simulink model "sedemo_preempt_policy"  (Simulink 7.5)
settings: Solver=VariableStepDiscrete  StartTime=0.0  StopTime=15  MaxStep=inf  RelTol=1e-3
libraries: simeventssink1 x10, simeventsgenerators1 x6, simeventsqueue1 x3, simeventsattributes2 x3, simeventsserver1 x3, simeventsprobes1 x2, simeventsrouting1 x2
settings Model: Creator=The MathWorks Inc.  ExtModeAutoUpdateStatusClock=off
settings DataIOCC: SaveOutput=off  SaveTime=off
settings OptimizationCC: InitFltsAndDblsToZero=on
settings DebuggingCC: AlgebraicLoopMsg=error  SaveWithParameterizedLinksMsg=none  SignalResolutionControl=TryResolveAllWithWarning  SolverPrmCheckMsg=none  MultiTaskDSMMsg=warning  MultiTaskCondExecSysMsg=none  StrictBusMsg=Warning
settings RTWCC: IncludeERTFirstTime=on
settings GRTTargetCC: TargetFcnLib=ansi_tfl_tmw.mat
settings SimEventsCC: propIdentEventSeed=12345678  propDiagAttribOutput=1  propDiagFcnCallOutput=1  propDiagStatOutput=0  propRNGIdenticalSeeds=0

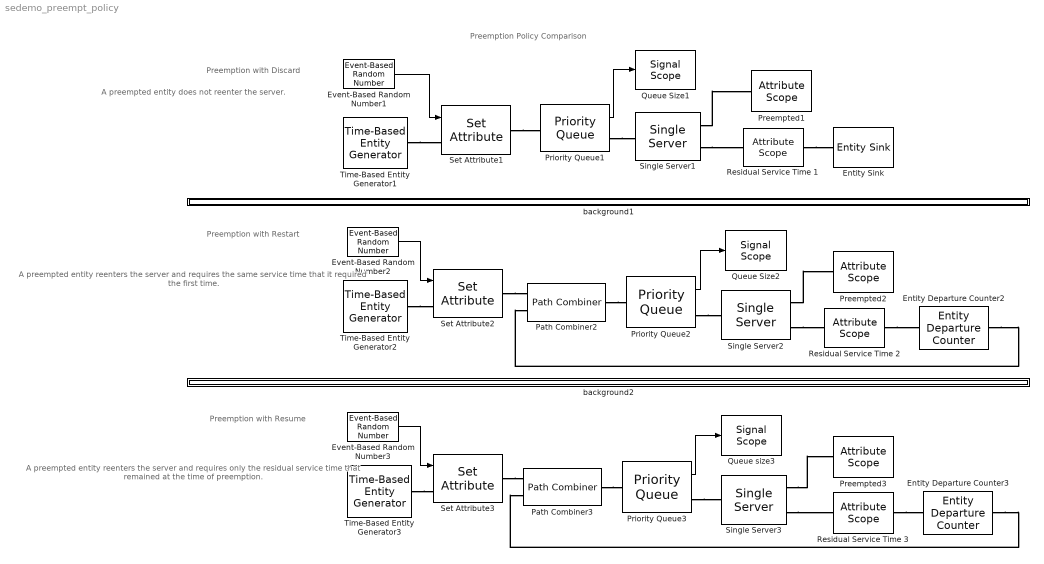
== system sedemo_preempt_policy ==
  note: Preemption with Restart
  note: Preemption with Resume
  note: A preempted entity does
      | not reenter the server.
  note: Preemption with Discard
  note: Preemption Policy Comparison
  note: A preempted entity reenters
      | the server and requires the
      | same service time that it
      | required the first time.
  note: A preempted entity reenters
      | the server and requires only
      | the residual service time
      | that remained at the time
      | of preemption.
  Entity Departure Counter2 : simeventsprobes1/Entity Departure Counter  Priority=1  SystemSampleTime=-1  NumberDepartedToSignal=Off  NumberDepartedToAttribute=On  NumberDepartedAttributeName=Preempted  CreateAttribute=on  CounterResetTypeOption=Off  CounterResetEdgeOption=Rising  SpecifyEventPriority=off  PriorityEntityCounterReset=1
  Entity Departure Counter3 : simeventsprobes1/Entity Departure Counter  Priority=1  SystemSampleTime=-1  NumberDepartedToSignal=Off  NumberDepartedToAttribute=On  NumberDepartedAttributeName=Preempted  CreateAttribute=on  CounterResetTypeOption=Off  CounterResetEdgeOption=Rising  SpecifyEventPriority=off  PriorityEntityCounterReset=1
  Entity Sink : simeventssink1/Entity Sink  Priority=1  SystemSampleTime=-1  AvailableForArrivals=on  StatNumberArrived=Off
  Event-Based Random Number1 : simeventsgenerators1/Signal Generators/Event-Based Random Number  SystemSampleTime=-1  distribution=Arbitrary discrete  meanExp=1  minUnif=0  maxUnif=1  pOneBern=0.25  pSuccessBino=0.5  numTrialBino=1  meanNorm=0  stdNorm=1  minTri=1  maxTri=3  modeTri=2  thresholdLogn=0  scaleLogn=1  shapeLogn=1  pSuccessGeo=0.5  meanPoiss=1  thresholdLogl=0  scaleLogl=1  thresholdGam=0  scaleGam=1  shapeGam=1  minBeta=0  maxBeta=1  shape1Beta=1  shape2Beta=1  minUnid=0  maxUnid=1  numValueUnid=2  thresholdWbl=0  scaleWbl=1  shapeWbl=1  valueVecCont=[0 1]  cdfVecCont=[0 1]  valueVecDisc=[1 2]  probVecDisc=[0.3 0.7]  seed=12345  IsProcessed=on  isConnected=1
  Event-Based Random Number2 : simeventsgenerators1/Signal Generators/Event-Based Random Number  SystemSampleTime=-1  distribution=Arbitrary discrete  meanExp=1  minUnif=0  maxUnif=1  pOneBern=0.25  pSuccessBino=0.5  numTrialBino=1  meanNorm=0  stdNorm=1  minTri=1  maxTri=3  modeTri=2  thresholdLogn=0  scaleLogn=1  shapeLogn=1  pSuccessGeo=0.5  meanPoiss=1  thresholdLogl=0  scaleLogl=1  thresholdGam=0  scaleGam=1  shapeGam=1  minBeta=0  maxBeta=1  shape1Beta=1  shape2Beta=1  minUnid=0  maxUnid=1  numValueUnid=2  thresholdWbl=0  scaleWbl=1  shapeWbl=1  valueVecCont=[0 1]  cdfVecCont=[0 1]  valueVecDisc=[1 2]  probVecDisc=[0.3 0.7]  seed=12345  IsProcessed=on  isConnected=1
  Event-Based Random Number3 : simeventsgenerators1/Signal Generators/Event-Based Random Number  SystemSampleTime=-1  distribution=Arbitrary discrete  meanExp=1  minUnif=0  maxUnif=1  pOneBern=0.25  pSuccessBino=0.5  numTrialBino=1  meanNorm=0  stdNorm=1  minTri=1  maxTri=3  modeTri=2  thresholdLogn=0  scaleLogn=1  shapeLogn=1  pSuccessGeo=0.5  meanPoiss=1  thresholdLogl=0  scaleLogl=1  thresholdGam=0  scaleGam=1  shapeGam=1  minBeta=0  maxBeta=1  shape1Beta=1  shape2Beta=1  minUnid=0  maxUnid=1  numValueUnid=2  thresholdWbl=0  scaleWbl=1  shapeWbl=1  valueVecCont=[0 1]  cdfVecCont=[0 1]  valueVecDisc=[1 2]  probVecDisc=[0.3 0.7]  seed=12345  IsProcessed=on  isConnected=1
  Path Combiner2 : simeventsrouting1/Path Combiner  Priority=1  SystemSampleTime=-1  NumberInputPorts=2  InputPortPrecedence=IN1 port  InitialSeed=45675  SpecifyEventPriority=off  PriorityPathCombinerPortPrecedenceSelection=4100  StatNumberDeparted=Off  StatLastArrivalPort=Off  EvaluatedNumPorts=2
  Path Combiner3 : simeventsrouting1/Path Combiner  Priority=1  SystemSampleTime=-1  NumberInputPorts=2  InputPortPrecedence=IN1 port  InitialSeed=45675  SpecifyEventPriority=off  PriorityPathCombinerPortPrecedenceSelection=4100  StatNumberDeparted=Off  StatLastArrivalPort=Off  EvaluatedNumPorts=2
  Preempted1 : simeventssink1/Attribute Scope  Priority=1  SystemSampleTime=-1  PlotType=Stem  InputType=Attribute  NumInputs=1  AttributeNameY=Preempted  XInputOptionSignal=Event time  XInputOptionEntity=Event time  AttributeNameX=Count  EnableEntityOutport=off  XMin=0  XMax=15  XLimitExceededOption=Stretch axis limits  YLimitExceededOption=Stretch axis limits  AxisGrid=on  AxisLegend=off  LineDisables=""  LineColors=b  LineStyles=-  LineMarkers=.  OpenScopeAtSimStart=on  Title=Discard Policy: Preempted  YLabel=Preempted  XLabel=Time  FigurePosition=[74 417 276 169]  AxisZoom=off  DataStoreOption=Limited  DataPointsLimit=10000  StatNumberArrived=Off  ShowCountPlotted=off  ShowToolbar=off
      settings: YMin=-2  YMax=2
  Preempted2 : simeventssink1/Attribute Scope  Priority=1  SystemSampleTime=-1  PlotType=Stem  InputType=Attribute  NumInputs=1  AttributeNameY=Preempted  XInputOptionSignal=Event time  XInputOptionEntity=Event time  AttributeNameX=Count  EnableEntityOutport=off  XMin=0  XMax=15  XLimitExceededOption=Stretch axis limits  YLimitExceededOption=Stretch axis limits  AxisGrid=on  AxisLegend=off  LineDisables=""  LineColors=b  LineStyles=-  LineMarkers=.  OpenScopeAtSimStart=on  Title=Restart Policy: Preempted  YLabel=Preempted  XLabel=Time  FigurePosition=[75 236 275 173]  AxisZoom=off  DataStoreOption=Limited  DataPointsLimit=10000  StatNumberArrived=Off  ShowCountPlotted=off  ShowToolbar=off
      settings: YMin=-2  YMax=2
  Preempted3 : simeventssink1/Attribute Scope  Priority=1  SystemSampleTime=-1  PlotType=Stem  InputType=Attribute  NumInputs=1  AttributeNameY=Preempted  XInputOptionSignal=Event time  XInputOptionEntity=Event time  AttributeNameX=Count  EnableEntityOutport=off  XMin=0  XMax=15  XLimitExceededOption=Stretch axis limits  YLimitExceededOption=Stretch axis limits  AxisGrid=on  AxisLegend=off  LineDisables=""  LineColors=b  LineStyles=-  LineMarkers=.  OpenScopeAtSimStart=on  Title=Resume Policy: Preempted  YLabel=Preempted  XLabel=Time  FigurePosition=[72 56 274 174]  AxisZoom=off  DataStoreOption=Limited  DataPointsLimit=10000  StatNumberArrived=Off  ShowCountPlotted=off  ShowToolbar=off
      settings: YMin=-2  YMax=2
  Priority Queue1 : simeventsqueue1/Priority Queue  Priority=1  SystemSampleTime=-1  Capacity=25  SortingAttributeName=PriorityAttributeName  SortingDirection=Ascending  EnableTOPort=off  StatNumberDeparted=Off  StatNumberInBlock=On  StatPendingEntity=Off  StatAverageWait=Off  StatAverageQueueLength=Off  StatNumberTimedout=Off
  Priority Queue2 : simeventsqueue1/Priority Queue  Priority=1  SystemSampleTime=-1  Capacity=25  SortingAttributeName=PriorityAttributeName  SortingDirection=Ascending  EnableTOPort=off  StatNumberDeparted=Off  StatNumberInBlock=On  StatPendingEntity=Off  StatAverageWait=Off  StatAverageQueueLength=Off  StatNumberTimedout=Off
  Priority Queue3 : simeventsqueue1/Priority Queue  Priority=1  SystemSampleTime=-1  Capacity=25  SortingAttributeName=PriorityAttributeName  SortingDirection=Ascending  EnableTOPort=off  StatNumberDeparted=Off  StatNumberInBlock=On  StatPendingEntity=Off  StatAverageWait=Off  StatAverageQueueLength=Off  StatNumberTimedout=Off
  Queue Size1 : simeventssink1/Signal Scope  Priority=1  SystemSampleTime=-1  PlotType=Stair  InputType=Signal  NumInputs=1  AttributeNameY=Count  XInputOptionSignal=Event time  XInputOptionEntity=Event time  AttributeNameX=Count  EnableEntityOutport=on  XMin=0  XMax=15  XLimitExceededOption=Stretch axis limits  YLimitExceededOption=Stretch axis limits  AxisGrid=on  AxisLegend=off  LineDisables=""  LineColors=b  LineStyles=-  LineMarkers=.  OpenScopeAtSimStart=on  Title=Discard Policy: Queue Size  YLabel=Queue Size  XLabel=Time  FigurePosition=[640 413 278 171]  AxisZoom=off  DataStoreOption=Limited  DataPointsLimit=10000  StatNumberArrived=Off  ShowCountPlotted=off  ShowToolbar=off
      settings: YMin=0  YMax=5
  Queue Size2 : simeventssink1/Signal Scope  Priority=1  SystemSampleTime=-1  PlotType=Stair  InputType=Signal  NumInputs=1  AttributeNameY=Count  XInputOptionSignal=Event time  XInputOptionEntity=Event time  AttributeNameX=Count  EnableEntityOutport=on  XMin=0  XMax=15  XLimitExceededOption=Stretch axis limits  YLimitExceededOption=Stretch axis limits  AxisGrid=on  AxisLegend=off  LineDisables=""  LineColors=b  LineStyles=-  LineMarkers=.  OpenScopeAtSimStart=on  Title=Restart Policy: Queue Size  YLabel=Queue Size  XLabel=Time  FigurePosition=[643 238 278 171]  AxisZoom=off  DataStoreOption=Limited  DataPointsLimit=10000  StatNumberArrived=Off  ShowCountPlotted=off  ShowToolbar=off
      settings: YMin=0  YMax=5
  Queue size3 : simeventssink1/Signal Scope  Priority=1  SystemSampleTime=-1  PlotType=Stair  InputType=Signal  NumInputs=1  AttributeNameY=Count  XInputOptionSignal=Event time  XInputOptionEntity=Event time  AttributeNameX=Count  EnableEntityOutport=on  XMin=0  XMax=15  XLimitExceededOption=Stretch axis limits  YLimitExceededOption=Stretch axis limits  AxisGrid=on  AxisLegend=off  LineDisables=""  LineColors=b  LineStyles=-  LineMarkers=.  OpenScopeAtSimStart=on  Title=Resume Policy: Queue Size  YLabel=Queue Size  XLabel=Time  FigurePosition=[640 56 278 171]  AxisZoom=off  DataStoreOption=Limited  DataPointsLimit=10000  StatNumberArrived=Off  ShowCountPlotted=off  ShowToolbar=off
      settings: YMin=0  YMax=5
  Residual Service Time 1 : simeventssink1/Attribute Scope  Priority=1  SystemSampleTime=-1  PlotType=Stair  InputType=Attribute  NumInputs=1  AttributeNameY=ResidualServiceTime  XInputOptionSignal=Event time  XInputOptionEntity=Event time  AttributeNameX=Count  EnableEntityOutport=on  XMin=0  XMax=15  XLimitExceededOption=Stretch axis limits  YLimitExceededOption=Stretch axis limits  AxisGrid=on  AxisLegend=off  LineDisables=""  LineColors=b  LineStyles=-  LineMarkers=.  OpenScopeAtSimStart=on  Title=Discard Policy: Residual Service Time  YLabel=Residual Service Time  XLabel=Time  FigurePosition=[357 413 290 176]  AxisZoom=off  DataStoreOption=Limited  DataPointsLimit=10000  StatNumberArrived=Off  ShowCountPlotted=off  ShowToolbar=off
      settings: YMin=0  YMax=2
  Residual Service Time 2 : simeventssink1/Attribute Scope  Priority=1  SystemSampleTime=-1  PlotType=Stair  InputType=Attribute  NumInputs=1  AttributeNameY=ResidualServiceTime  XInputOptionSignal=Event time  XInputOptionEntity=Event time  AttributeNameX=Count  EnableEntityOutport=on  XMin=0  XMax=15  XLimitExceededOption=Stretch axis limits  YLimitExceededOption=Stretch axis limits  AxisGrid=on  AxisLegend=off  LineDisables=""  LineColors=b  LineStyles=-  LineMarkers=.  OpenScopeAtSimStart=on  Title=Restart Policy: Residual Service Time  YLabel=Residual Service Time  XLabel=Time  FigurePosition=[356 235 280 170]  AxisZoom=off  DataStoreOption=Limited  DataPointsLimit=10000  StatNumberArrived=Off  ShowCountPlotted=off  ShowToolbar=off
      settings: YMin=0  YMax=2
  Residual Service Time 3 : simeventssink1/Attribute Scope  Priority=1  SystemSampleTime=-1  PlotType=Stair  InputType=Attribute  NumInputs=1  AttributeNameY=ServiceTime  XInputOptionSignal=Event time  XInputOptionEntity=Event time  AttributeNameX=Count  EnableEntityOutport=on  XMin=0  XMax=15  XLimitExceededOption=Stretch axis limits  YLimitExceededOption=Stretch axis limits  AxisGrid=on  AxisLegend=off  LineDisables=""  LineColors=b  LineStyles=-  LineMarkers=.  OpenScopeAtSimStart=on  Title=Resume Policy: Residual Service Time  YLabel=Residual Service Time  XLabel=Time  FigurePosition=[357 56 279 169]  AxisZoom=off  DataStoreOption=Limited  DataPointsLimit=10000  StatNumberArrived=Off  ShowCountPlotted=off  ShowToolbar=off
      settings: YMin=0  YMax=2
  Set Attribute1 : simeventsattributes2/Set Attribute  Priority=1  DialogController=des_ddg_create  DialogControllerArgs=DataTag18  SystemSampleTime=-1  AttributeFrom=Signal port|Dialog|Dialog  AttributeName=PriorityAttributeName|ServiceTime|Preempted  AttributeTreatAsVector=1|1|1  AttributeValue=1|1.2|-1  AttributeCreate=on  StatNumberDeparted=Off  EvaluatedAttributeValue={[];1.2;-1}
  Set Attribute2 : simeventsattributes2/Set Attribute  Priority=1  DialogController=des_ddg_create  DialogControllerArgs=DataTag20  SystemSampleTime=-1  AttributeFrom=Signal port|Dialog|Dialog  AttributeName=PriorityAttributeName|ServiceTime|Preempted  AttributeTreatAsVector=1|1|1  AttributeValue=1|1.2|-1  AttributeCreate=on  StatNumberDeparted=Off  EvaluatedAttributeValue={[];1.2;-1}
  Set Attribute3 : simeventsattributes2/Set Attribute  Priority=1  DialogController=des_ddg_create  DialogControllerArgs=DataTag22  SystemSampleTime=-1  AttributeFrom=Signal port|Dialog|Dialog  AttributeName=PriorityAttributeName|ServiceTime|Preempted  AttributeTreatAsVector=1|1|1  AttributeValue=1|1.2|-1  AttributeCreate=on  StatNumberDeparted=Off  EvaluatedAttributeValue={[];1.2;-1}
  Single Server1 : simeventsserver1/Single Server  Priority=1  SystemSampleTime=-1  ServiceTimeFrom=Attribute  ServiceTime=1.2  AttributeName=ServiceTime  PriorityServiceCompletion=50  PermitPreemption=on  SortingAttributeName=PriorityAttributeName  SortingDirection=Ascending  WriteToAttribute=on  ResidualAttributeName=ResidualServiceTime  CreateAttribute=on  EnableTOPort=off  StatNumberDeparted=Off  StatNumberInBlock=Off  StatNumberPreempted=Off  StatPendingEntity=Off  StatAverageWait=Off  StatUtilization=Off  StatNumberTimedout=Off
  Single Server2 : simeventsserver1/Single Server  Priority=1  SystemSampleTime=-1  ServiceTimeFrom=Attribute  ServiceTime=1.2  AttributeName=ServiceTime  PriorityServiceCompletion=50  PermitPreemption=on  SortingAttributeName=PriorityAttributeName  SortingDirection=Ascending  WriteToAttribute=on  ResidualAttributeName=ResidualServiceTime  CreateAttribute=on  EnableTOPort=off  StatNumberDeparted=Off  StatNumberInBlock=Off  StatNumberPreempted=Off  StatPendingEntity=Off  StatAverageWait=Off  StatUtilization=Off  StatNumberTimedout=Off
  Single Server3 : simeventsserver1/Single Server  Priority=1  SystemSampleTime=-1  ServiceTimeFrom=Attribute  ServiceTime=1.2  AttributeName=ServiceTime  PriorityServiceCompletion=50  PermitPreemption=on  SortingAttributeName=PriorityAttributeName  SortingDirection=Ascending  WriteToAttribute=on  ResidualAttributeName=ServiceTime  CreateAttribute=on  EnableTOPort=off  StatNumberDeparted=Off  StatNumberInBlock=Off  StatNumberPreempted=Off  StatPendingEntity=Off  StatAverageWait=Off  StatUtilization=Off  StatNumberTimedout=Off
  Time-Based Entity Generator1 : simeventsgenerators1/Entity Generators/Time-Based Entity Generator  Priority=1  DialogController=des_ddg_create  DialogControllerArgs=DataTag27  SystemSampleTime=-1  GenerateEntitiesUpon=Intergeneration time from dialog  Distribution=Constant  Minimum=0  Maximum=1  Mean=1  InitialSeed=12345  Period=1  PriorityEntityGeneration=10  GenerateEntityAtSimulationStart=on  ResponseWhenBlocked=Error  ResponseWhenUnblocked=Immediate restart  EntityType=Standard  StatNumberDeparted=Off  StatPendingEntity=Off  StatAverageIntergenerationTime=Off
  Time-Based Entity Generator2 : simeventsgenerators1/Entity Generators/Time-Based Entity Generator  Priority=1  DialogController=des_ddg_create  DialogControllerArgs=DataTag29  SystemSampleTime=-1  GenerateEntitiesUpon=Intergeneration time from dialog  Distribution=Constant  Minimum=0  Maximum=1  Mean=1  InitialSeed=12345  Period=1  PriorityEntityGeneration=10  GenerateEntityAtSimulationStart=on  ResponseWhenBlocked=Error  ResponseWhenUnblocked=Immediate restart  EntityType=Standard  StatNumberDeparted=Off  StatPendingEntity=Off  StatAverageIntergenerationTime=Off
  Time-Based Entity Generator3 : simeventsgenerators1/Entity Generators/Time-Based Entity Generator  Priority=1  DialogController=des_ddg_create  DialogControllerArgs=DataTag31  SystemSampleTime=-1  GenerateEntitiesUpon=Intergeneration time from dialog  Distribution=Constant  Minimum=0  Maximum=1  Mean=1  InitialSeed=12345  Period=1  PriorityEntityGeneration=10  GenerateEntityAtSimulationStart=on  ResponseWhenBlocked=Error  ResponseWhenUnblocked=Immediate restart  EntityType=Standard  StatNumberDeparted=Off  StatPendingEntity=Off  StatAverageIntergenerationTime=Off
  background1 : Subsystem
      mask Display: disp('')
  background2 : Subsystem
      mask Display: disp('')
  wires:
  Event-Based Random Number2/1 -> Set Attribute2/1
  Priority Queue2/1 -> Queue Size2/1
  Event-Based Random Number3/1 -> Set Attribute3/1
  Priority Queue3/1 -> Queue size3/1
  Event-Based Random Number1/1 -> Set Attribute1/1
  Priority Queue1/1 -> Queue Size1/1
  connections:
  Time-Based Entity Generator2/RConn1 -- Set Attribute2/LConn1
  Single Server2/RConn1 -- Preempted2/LConn1
  Priority Queue2/RConn1 -- Single Server2/LConn1
  Path Combiner2/RConn1 -- Priority Queue2/LConn1
  Set Attribute2/RConn1 -- Path Combiner2/LConn1
  Single Server2/RConn2 -- Residual Service Time 2/LConn1
  Time-Based Entity Generator3/RConn1 -- Set Attribute3/LConn1
  Single Server3/RConn1 -- Preempted3/LConn1
  Priority Queue3/RConn1 -- Single Server3/LConn1
  Path Combiner3/RConn1 -- Priority Queue3/LConn1
  Set Attribute3/RConn1 -- Path Combiner3/LConn1
  Single Server3/RConn2 -- Residual Service Time 3/LConn1
  Residual Service Time 3/RConn1 -- Entity Departure Counter3/LConn1
  Entity Departure Counter3/RConn1 -- Path Combiner3/LConn2
  Residual Service Time 2/RConn1 -- Entity Departure Counter2/LConn1
  Entity Departure Counter2/RConn1 -- Path Combiner2/LConn2
  Time-Based Entity Generator1/RConn1 -- Set Attribute1/LConn1
  Single Server1/RConn1 -- Preempted1/LConn1
  Priority Queue1/RConn1 -- Single Server1/LConn1
  Set Attribute1/RConn1 -- Priority Queue1/LConn1
  Single Server1/RConn2 -- Residual Service Time 1/LConn1
  Residual Service Time 1/RConn1 -- Entity Sink/LConn1

== system sedemo_preempt_policy/background1 ==

== system sedemo_preempt_policy/background2 ==
